simulink model "Mixer_stream_Ex2"  (R2023a)
settings: Solver=VariableStepAuto  StartTime=0.0  StopTime=1  RelTol=1e-3
undefined symbols (not defined in the file): None, S, vsva2197, xcvc1902
libraries: aieUtilities x8, dspsrcs4 x2, aieDSP x1, dspsigops x1, vmcUtilities x1
settings Model: Creator=sdegala  LastModifiedBy=robg
settings ModelReferenceCC: EnableRefExpFcnMdlSchedulingChecks=on

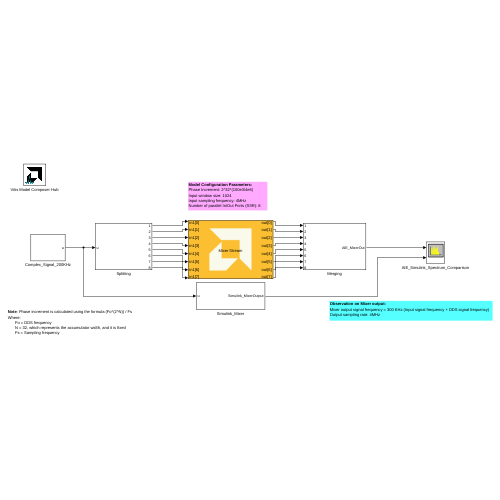
[thumbnail: Simulink's stored preview of the top-level diagram]
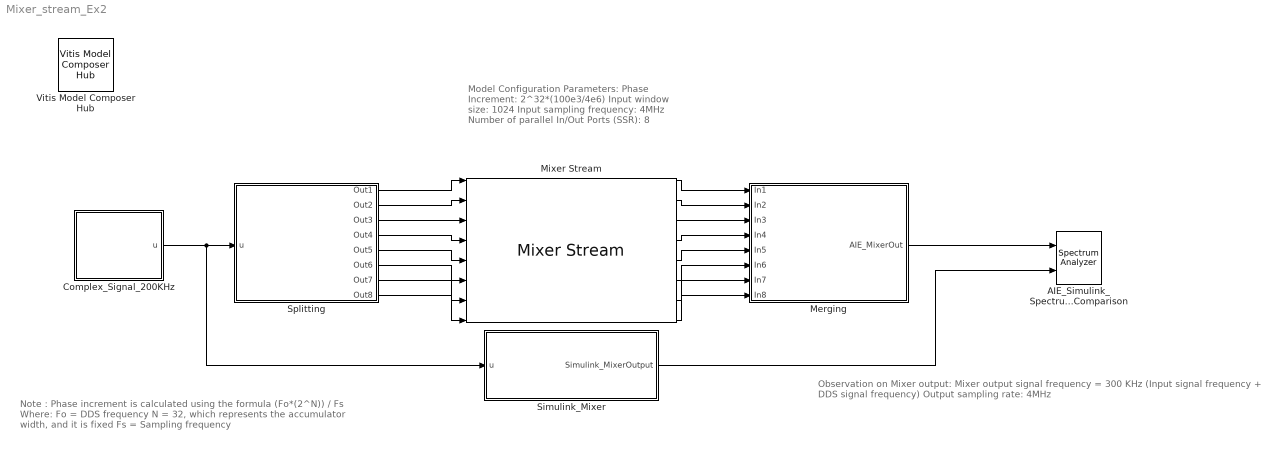
== system Mixer_stream_Ex2 ==
  note: Note : Phase increment is calculated using the formula (Fo*(2^N)) / Fs
      | Where:
      | Fo = DDS frequency
      | N = 32, which represents the accumulator width, and it is fixed
      | Fs = Sampling frequency
  note: Model Configuration Parameters:
      | Phase Increment: 2^32*(100e3/4e6)
      | Input window size: 1024
      | Input sampling frequency: 4MHz
      | Number of parallel In/Out Ports (SSR): 8
  note: Observation on Mixer output:
      | Mixer output signal frequency = 300 KHz (Input signal frequency + DDS signal frequency)
      | Output sampling rate: 4MHz
  AIE_Simulink_Spectrum_Comparison : SpectrumAnalyzer  NumInputPorts=2  AveragingMethod=Exponential  ShowLegend=on  ChannelNames="[\"\"]"  DefaultConfigurationName=spbscopes.SpectrumAnalyzerBlockCfg
  Complex_Signal_200KHz : Subsystem
  Merging : Subsystem
  Mixer Stream : aieDSP/Mixer Stream  data_type=cfloat  input_window_size=1024  mixer_mode=Single Input Mode  ssr=8  rnd_mode=Round to positive infinity  sat_mode=0-None  phase_increment=1.0737e+08  USE_PHASE_RELOAD=off  initial_phase_offset=0  AIE_VARIANT=1  blockJsonConstraints=[]  blockJsonConstraintsInternal=[]  spec=vmc_stream_mixer.json  SerializedMaskParamNames=[]  SerializedMaskParamValues=[]  SerializedMaskParamVisibilities=[]  block_type=Mixer Stream  SerializedMaskParamDataypes=typename|uint|uint|uint|uint|uint|uint|bool|uint|uint  SerializedMaskParamEnumStrArr=0|0|Single Input Mode,Dual Input Mode|0|Floor,Ceiling,Round to positive infinity,Round to negative infinity,Round symmetrical to infinity,Round symmetrical to zero,Round convergent to even,Round convergent to odd|0-None,1-Asymmetric,3-Symmetric|0|0|0|0  SerializedMaskParamEnumValArr=0|0|1,2|0|0,1,2,3,4,5,6,7|0,1,3|0|0|0|0  SerializedMaskParamVectorArr=0|0|0|0|0|0|0|0|0|0
  Simulink_Mixer : Subsystem
  Splitting : Subsystem
  Vitis Model Composer Hub : vmcUtilities/Vitis Model Composer Hub  Tag=genX  CodeGeneration=off  StartColumn=1  NumberOfColumns=1  TargetDirectory=./code  exportDesign=off  analyzeDesign=off  validateDesignOnHw=off  ExportType=AI Engines  IpVendor=xilinx.com  IpLibrary=hls  IpVersion=1.0  IpHWLanguage=Verilog  AieCompilerOptions={}  AieSimulatorOptions={}  CreateTestbench=off  TestbenchStackSize=10  RunRtlSim=off  RunCSim=off  RunAieSim=off  AieSimTimeout=50000  RunAieSimProfiling=off  LaunchVitisAnalyzer=off  PlotOutput=off  RunX86Sim=off  X86SimTimeout=10  GenHwImage=off  GenLibadfXo=off  GenHwValidationCode=off  PlatformType=Not Specified  HwSystemType=Baremetal  HwValidationTarget=hw  ProjDevice=xcvc1902-vsva2197-1LP-e-S  ProjDevicePart=xcvc1902-vsva2197-1LP-e-S  AIEType=AIE  SamplePeriod=-1  ClockFrequency=200  DataPathParallelism=1  xilinxfamily=versalaicore  part=xcvc1902  speed=-1LP-e-S  package=vsva2197  directory=./netlist  testbench=off  incr_netlist=off  synthesis_tool=Vivado  clock_wrapper=Clock Enables  dbl_ovrd=According to Block Masks  dcm_input_clock_period=10  sysclk_period=10  simulink_period=1  eval_field=0  LogFileName=''  NThreads=4
  wires:
  Simulink_Mixer/1(Simulink_MixerOutput) -> AIE_Simulink_Spectrum_Comparison/2
  Complex_Signal_200KHz/1(u) -> Simulink_Mixer/1(u), Splitting/1(u)
  Merging/1(AIE_MixerOut) -> AIE_Simulink_Spectrum_Comparison/1
  Splitting/1(Out1) -> Mixer Stream/1
  Splitting/2(Out2) -> Mixer Stream/2
  Splitting/3(Out3) -> Mixer Stream/3
  Splitting/4(Out4) -> Mixer Stream/4
  Splitting/5(Out5) -> Mixer Stream/5
  Splitting/6(Out6) -> Mixer Stream/6
  Splitting/7(Out7) -> Mixer Stream/7
  Splitting/8(Out8) -> Mixer Stream/8
  Mixer Stream/1 -> Merging/1(In1)
  Mixer Stream/2 -> Merging/2(In2)
  Mixer Stream/3 -> Merging/3(In3)
  Mixer Stream/4 -> Merging/4(In4)
  Mixer Stream/5 -> Merging/5(In5)
  Mixer Stream/6 -> Merging/6(In6)
  Mixer Stream/7 -> Merging/7(In7)
  Mixer Stream/8 -> Merging/8(In8)

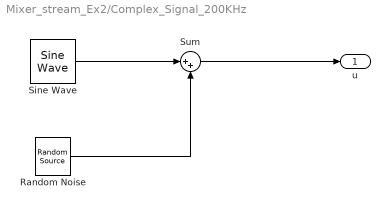
== system Mixer_stream_Ex2/Complex_Signal_200KHz ==
  Random Noise : dspsrcs4/Random Source  SrcType=Gaussian  NormMethod=Ziggurat  CltLength=12  MinVal=0  MaxVal=1  MeanVal=0  VarVal=1e-3  RepMode=Not repeatable  rawSeed=1  IsInherit=off  SampMode=Discrete  SampTime=1/4e6  SampFrame=1024  DataType=Single  OutComplex=Real  OutputFrames=off
  Sine Wave : dspsrcs4/Sine Wave  Amplitude=1  Frequency=200e3  Phase=0  SampleMode=Discrete  OutComplex=Complex  CompMethod=Trigonometric fcn  TableSize=Speed  SampleTime=1/4e6  SamplesPerFrame=1024  ResetState=Restart at time zero  OutputFrames=off  dataType=single  wordLen=16  udDataType=sfix(16)  fracBitsMode=Best precision  numFracBits=15  OutDataTypeStr=single  LastOutDataTypeStr=single
  Sum : Sum  Inputs=|++
  u : Outport
  wires:
  Sine Wave/1 -> Sum/1
  Sum/1 -> u/1
  Random Noise/1 -> Sum/2

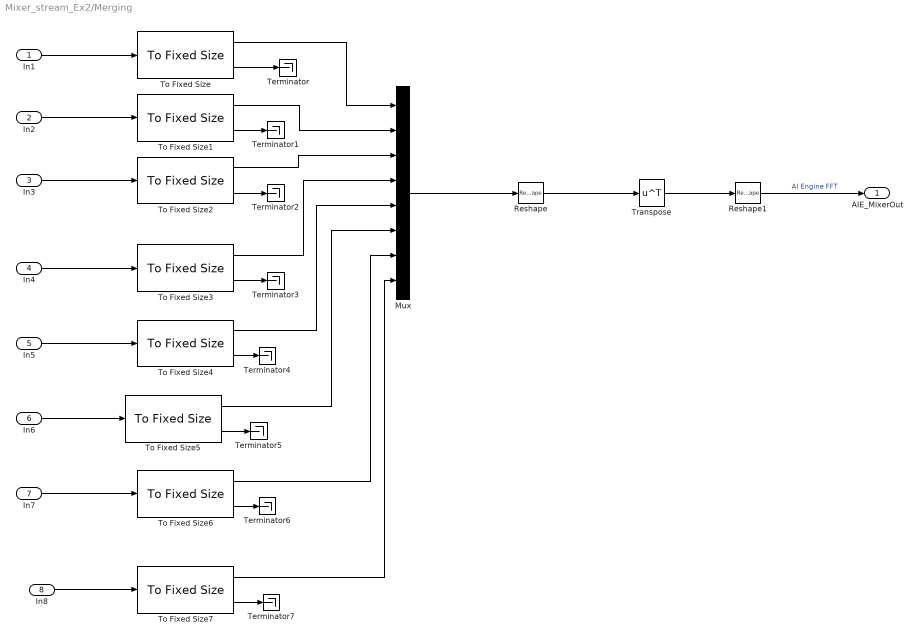
== system Mixer_stream_Ex2/Merging ==
  In1 : Inport
  In2 : Inport  Port=2
  In3 : Inport  Port=3
  In4 : Inport  Port=4
  In5 : Inport  Port=5
  In6 : Inport  Port=6
  In7 : Inport  Port=7
  In8 : Inport  Port=8
  Mux : Mux  Inputs=8
  Reshape : Reshape  OutputDimensionality=Customize  OutputDimensions=[128, 8]
  Reshape1 : Reshape  OutputDimensions=[1, 10]
  Terminator{,1..7} (8 alike) : Terminator
  To Fixed Size{,1..7} (8 alike) : aieUtilities/To Fixed Size  Mode=Produce a valid output signal  OutputSize=Inherit: Same as input  CopyMethod=Buffer samples to form output  HasStatusOutput=on
  Transpose : Math  Operator=transpose
  AIE_MixerOut : Outport
  wires:
  Reshape/1 -> Transpose/1
  To Fixed Size1/2 -> Terminator1/1
  To Fixed Size1/1 -> Mux/2
  In2/1 -> To Fixed Size1/1
  To Fixed Size/2 -> Terminator/1
  Transpose/1 -> Reshape1/1
  To Fixed Size/1 -> Mux/1
  Mux/1 -> Reshape/1
  Reshape1/1 -> AIE_MixerOut/1  "AI Engine FFT"
  In1/1 -> To Fixed Size/1
  To Fixed Size2/2 -> Terminator2/1
  In4/1 -> To Fixed Size3/1
  To Fixed Size3/1 -> Mux/4
  To Fixed Size3/2 -> Terminator3/1
  In3/1 -> To Fixed Size2/1
  To Fixed Size2/1 -> Mux/3
  To Fixed Size4/2 -> Terminator4/1
  In6/1 -> To Fixed Size5/1
  To Fixed Size5/2 -> Terminator5/1
  In5/1 -> To Fixed Size4/1
  To Fixed Size5/1 -> Mux/6
  To Fixed Size4/1 -> Mux/5
  To Fixed Size7/1 -> Mux/8
  To Fixed Size6/1 -> Mux/7
  In7/1 -> To Fixed Size6/1
  In8/1 -> To Fixed Size7/1
  To Fixed Size6/2 -> Terminator6/1
  To Fixed Size7/2 -> Terminator7/1

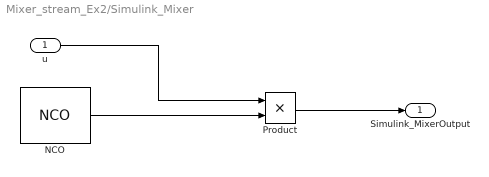
== system Mixer_stream_Ex2/Simulink_Mixer ==
  u : Inport
  NCO : dspsigops/NCO  AccIncSrc=Specify via dialog  AccInc=1.0737e+08  PhaseOffsetSrc=Specify via dialog  PhaseOffset=0  AccumWL=32  HasDither=off  DitherWL=4  PNgeneratorLength=19  HasPhaseQuantizer=on  TableDepth=16  HasOutputPhaseError=off  Formula=Complex exponential  DataType=single  OutputWL=16  OutputFL=14  CompMethod=Table lookup (no interpolation)  SampleTime=1/4e6  SamplesPerFrame=1024  OutputFrames=off
  Product : Product
  Simulink_MixerOutput : Outport
  wires:
  NCO/1 -> Product/2
  u/1 -> Product/1
  Product/1 -> Simulink_MixerOutput/1

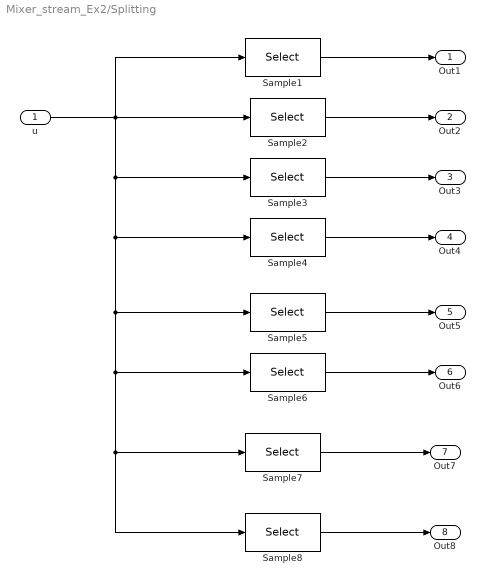
== system Mixer_stream_Ex2/Splitting ==
  u : Inport
  Sample1 : Selector  InputPortWidth=1024  IndexOptions=Index vector (dialog)  Indices=1:8:1024  OutputSizes=1
  Sample2 : Selector  InputPortWidth=1024  IndexOptions=Index vector (dialog)  Indices=2:8:1024  OutputSizes=1
  Sample3 : Selector  InputPortWidth=1024  IndexOptions=Index vector (dialog)  Indices=3:8:1024  OutputSizes=1
  Sample4 : Selector  InputPortWidth=1024  IndexOptions=Index vector (dialog)  Indices=4:8:1024  OutputSizes=1
  Sample5 : Selector  InputPortWidth=1024  IndexOptions=Index vector (dialog)  Indices=5:8:1024  OutputSizes=1
  Sample6 : Selector  InputPortWidth=1024  IndexOptions=Index vector (dialog)  Indices=6:8:1024  OutputSizes=1
  Sample7 : Selector  InputPortWidth=1024  IndexOptions=Index vector (dialog)  Indices=7:8:1024  OutputSizes=1
  Sample8 : Selector  InputPortWidth=1024  IndexOptions=Index vector (dialog)  Indices=8:8:1024  OutputSizes=1
  Out1 : Outport
  Out2 : Outport  Port=2
  Out3 : Outport  Port=3
  Out4 : Outport  Port=4
  Out5 : Outport  Port=5
  Out6 : Outport  Port=6
  Out7 : Outport  Port=7
  Out8 : Outport  Port=8
  wires:
  Sample2/1 -> Out2/1
  Sample1/1 -> Out1/1
  Sample3/1 -> Out3/1
  Sample4/1 -> Out4/1
  Sample5/1 -> Out5/1
  Sample6/1 -> Out6/1
  u/1 -> Sample5/1, Sample8/1, Sample7/1, Sample6/1, Sample4/1, Sample3/1, Sample2/1, Sample1/1
  Sample7/1 -> Out7/1
  Sample8/1 -> Out8/1
